simulink model "UAV01_step1"  (R2025a)
settings: Solver=VariableStepAuto  StartTime=0.0  StopTime=10.0  RelTol=1e-3
settings Model: Creator=ayeo  LastModifiedBy=ayeo

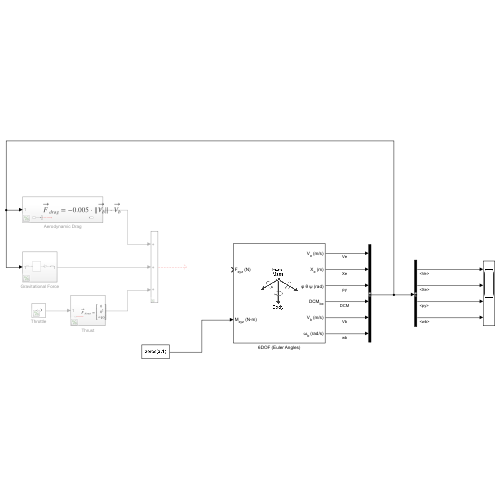
[thumbnail: Simulink's stored preview of the top-level diagram]
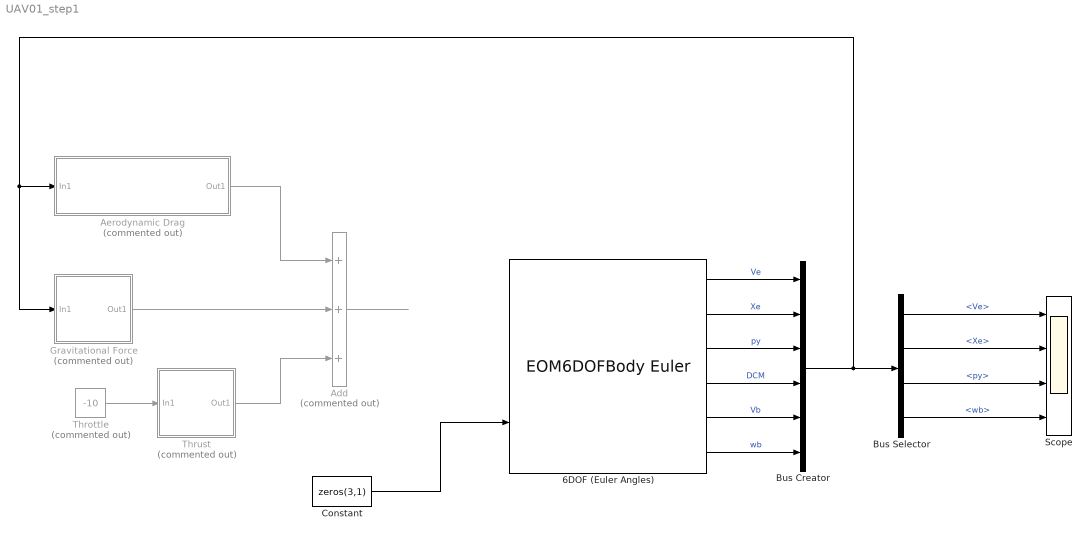
== system UAV01_step1 ==
  6DOF (Euler Angles) : EOM6DOFBodyEuler
  Add : Sum  Commented=on  Inputs=+++
  Aerodynamic Drag : Subsystem  Commented=on
  Bus Creator : BusCreator  Inputs=6
  Bus Selector : BusSelector  OutputSignals=Ve,Xe,py,wb
  Constant : Constant  Value=zeros(3,1)
  Gravitational Force : Subsystem  Commented=on
  Scope : Scope  NumInputPorts=4
  Throttle : Constant  Commented=on  Value=-10
  Thrust : Subsystem  Commented=on
  wires:
  Constant/1 -> 6DOF (Euler Angles)/2
  6DOF (Euler Angles)/1 -> Bus Creator/1  "Ve"
  6DOF (Euler Angles)/3 -> Bus Creator/3  "py"
  6DOF (Euler Angles)/2 -> Bus Creator/2  "Xe"
  6DOF (Euler Angles)/4 -> Bus Creator/4  "DCM"
  6DOF (Euler Angles)/5 -> Bus Creator/5  "Vb"
  6DOF (Euler Angles)/6 -> Bus Creator/6  "wb"
  Bus Selector/1 -> Scope/1  "<Ve>"
  Bus Selector/2 -> Scope/2  "<Xe>"
  Bus Selector/3 -> Scope/3  "<py>"
  Bus Selector/4 -> Scope/4  "<wb>"
  Bus Creator/1 -> Aerodynamic Drag/1(In1), Gravitational Force/1(In1), Bus Selector/1
  Throttle/1 -> Thrust/1(In1)
  Aerodynamic Drag/1(Out1) -> Add/1
  Add/1 -> ?
  Gravitational Force/1(Out1) -> Add/2
  Thrust/1(Out1) -> Add/3

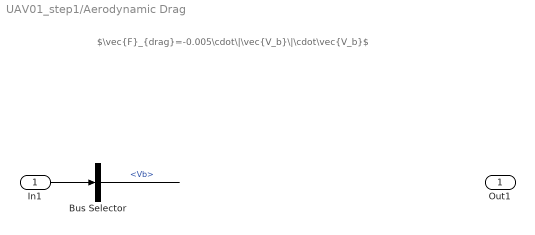
== system UAV01_step1/Aerodynamic Drag ==
  note: $\vec{F}_{drag}=-0.005\cdot\|\vec{V_b}\|\cdot\vec{V_b}$
  In1 : Inport
  Bus Selector : BusSelector  OutputSignals=Vb
  Out1 : Outport
  wires:
  In1/1 -> Bus Selector/1
  Bus Selector/1 -> ?  "<Vb>"

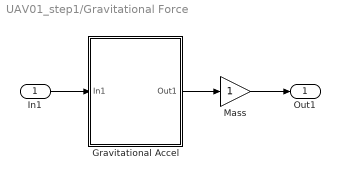
== system UAV01_step1/Gravitational Force ==
  In1 : Inport
  Gravitational Accel : Subsystem
  Mass : Gain
  Out1 : Outport
  wires:
  Gravitational Accel/1(Out1) -> Mass/1
  In1/1 -> Gravitational Accel/1(In1)
  Mass/1 -> Out1/1

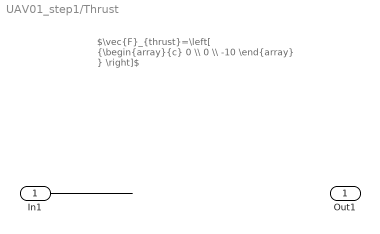
== system UAV01_step1/Thrust ==
  note: $\vec{F}_{thrust}=\left[ {\begin{array}{c} 0 \\ 0 \\ -10 \end{array} } \right]$
  In1 : Inport
  Out1 : Outport
  wires:
  In1/1 -> ?

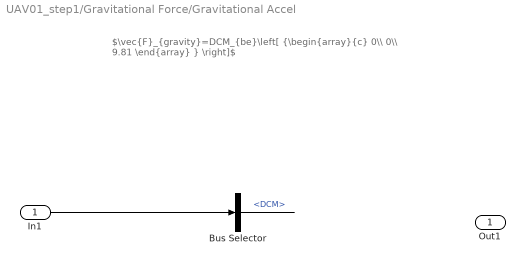
== system UAV01_step1/Gravitational Force/Gravitational Accel ==
  note: $\vec{F}_{gravity}=DCM_{be}\left[ {\begin{array}{c} 0\\ 0\\ 9.81 \end{array} } \right]$
  In1 : Inport
  Bus Selector : BusSelector  OutputSignals=DCM
  Out1 : Outport
  wires:
  In1/1 -> Bus Selector/1
  Bus Selector/1 -> ?  "<DCM>"
